simulink model "PuzzleMark5"  (R2022b)
settings: Solver=FixedStepAuto  StartTime=0.0  StopTime=160  FixedStep=0.001  RelTol=1e-3
libraries: slpidlib x2
settings Model: Creator=betel  LastModifiedBy=ivan
settings OptimizationCC: ReuseModelBlockBuffer=on

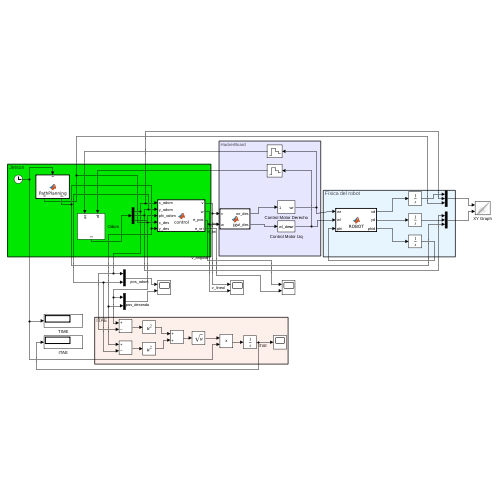
[thumbnail: Simulink's stored preview of the top-level diagram]
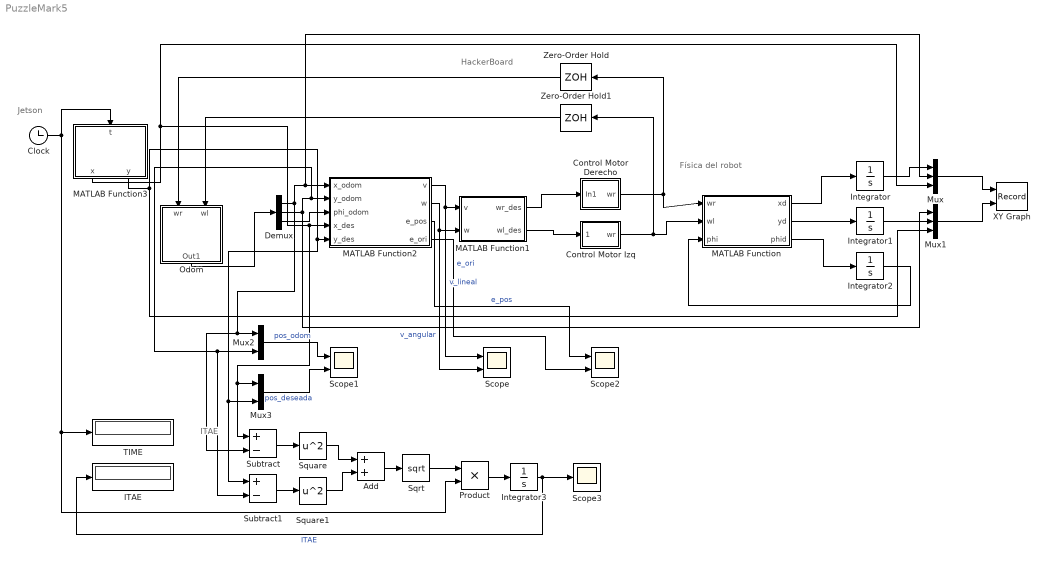
== system PuzzleMark5 ==
  note: ITAE
  note: Jetson
  note: Física del robot
  note: HackerBoard
  Add : Sum
  Clock : Clock
  Control Motor Derecho : Subsystem
  Control Motor Izq : Subsystem
  Demux : Demux  Outputs=3
  ITAE : Display
  Integrator : Integrator  ContinuousStateAttributes='x'
  Integrator1 : Integrator  ContinuousStateAttributes='y'
  Integrator2 : Integrator  ContinuousStateAttributes='orientation'
  Integrator3 : Integrator
  MATLAB Function : MATLAB Function  TreatAsAtomicUnit=on
  MATLAB Function1 : MATLAB Function  TreatAsAtomicUnit=on
  MATLAB Function2 : MATLAB Function  TreatAsAtomicUnit=on
  MATLAB Function3 : MATLAB Function  TreatAsAtomicUnit=on
  Mux : Mux  Inputs=3
  Mux1 : Mux  Inputs=3
  Mux2 : Mux  Inputs=2
  Mux3 : Mux  Inputs=2
  Odom : Subsystem
  Product : Product
  Scope : Scope  NumInputPorts=2
  Scope1 : Scope  NumInputPorts=2
  Scope2 : Scope  NumInputPorts=2
  Scope3 : Scope
  Sqrt : Sqrt
  Square : Math  Operator=square
  Square1 : Math  Operator=square
  Subtract : Sum  Inputs=+-
  Subtract1 : Sum  Inputs=+-
  TIME : Display
  XY Graph : Record  FileSettingsInternal="{\"entries\":[{\"content\":{\"excelSettings\":{\"content\":{},\"type\":\"Streamout.ExcelSettings\"}},\"type\":\"Streamout.FileSettingStorage\",\"uuid\":\"\"}],\"packageUris\":[\"http:\\/\\/schema.mathworks.com\\/mf0\\/streamout_blocks\\/R2020a\"],\"version\":\"1.0\"}"  Layout=[1 1]  SignalsInternal="{\"entries\":[{\"content\":{\"signals\":[{\"content\":{\"blockPath\":[],\"dimensions\":[3],\"domain\":\"\",\"hasChildren\":true,\"lineColor\":\"#77ac30\",\"lineWidth\":2,\"port\":1,\"signalID\":1,\"signalName\":\"Mux\"},\"type\":\"RecordBlkView.Signal\",\"uuid\":\"\"},{\"content\":{\"blockPath\":[],\"channel\":[1],\"dimensions\":[3],\"domain\":\"\",\"lineColor\":\"#139fff\",\"parentID\":1,\"plots\":[ 1 ],\"port\":1,\"signalID\":2,\"signalName\":\"Mux\"},\"type\":\"RecordBlkView.Signal\",\"uuid\":\"\"},{\"content\":{\"blockPath\":[],\"channel\":[2],\"dimensions\":[3],\"domain\":\"\",\"lineColor\":\"#64d413\",\"parentID\":1,\"plots\":[ 1 ],\"port\":1,\"signalID\":3,\"signalName\":\"Mux\"},\"type\":\"RecordBlkView.Signal\",\"uuid\":\"\"},{\"content\":{\"blockPath\":[],\"channel\":[3],\"dimensions\":[3],\"domain\":\"\",\"lineColor\":\"#4dbeee\",\"parentID\":1,\"plots\":[ 1 ],\"port\":1,\"signalID\":4,\"signalName\":\"Mux\"},\"type\":\"RecordBlkView.Signal\",\"uuid\":\"\"},{\"content\":{\"blockPath\":[],\"dimensions\":[3],\"domain\":\"\",\"hasChildren\":true,\"lineColor\":\"#a2142f\",\"lineWidth\":2,\"port\":2,\"signalID\":5,\"signalName\":\"Mux1\"},\"type\":\"RecordBlkView.Signal\",\"uuid\":\"\"},{\"content\":{\"blockPath\":[],\"channel\":[1],\"dimensions\":[3],\"domain\":\"\",\"lineColor\":\"#b746ff\",\"parentID\":5,\"plots\":[ 1 ],\"port\":2,\"signalID\":6,\"signalName\":\"Mux1\"},\"type\":\"RecordBlkView.Signal\",\"uuid\":\"\"},{\"content\":{\"blockPath\":[],\"channel\":[2],\"dimensions\":[3],\"domain\":\"\",\"lineColor\":\"#ff13a6\",\"parentID\":5,\"plots\":[ 1 ],\"port\":2,\"signalID\":7,\"signalName\":\"Mux1\"},\"type\":\"RecordBlkView.Signal\",\"uuid\":\"\"},{\"content\":{\"blockPath\":[],\"channel\":[3],\"dimensions\":[3],\"domain\":\"\",\"lineColor\":\"#fe330a\",\"parentID\":5,\"plots\":[ 1 ],\"port\":2,\"signalID\":8,\"signalName\":\"Mux1\"},\"type\":\"RecordBlkView.Signal\",\"uuid\":\"\"}]},\"type\":\"RecordBlkView.InputSignals\",\"uuid\":\"\"}],\"packageUris\":[\"http:\\/\\/schema.mathworks.com\\/mf0\\/streamout_blocks\\/R2020a\"],\"version\":\"1.0\"}"  VisualizationBindings="{\"xyplotplugin\":{\"info\":[{\"series\":[{\"bindingParametersList\":[{\"parameter\":\"X-Axis\",\"signalID\":2,\"signalName\":\"Mux(1)\"},{\"parameter\":\"Y-Axis\",\"signalID\":6,\"signalName\":\"Mux1(1)\"}],\"seriesID\":0},{\"bindingParametersList\":[{\"parameter\":\"X-Axis\",\"signalID\":3,\"signalName\":\"Mux(2)\"},{\"parameter\":\"Y-Axis\",\"signalID\":7,\"signalName\":\"Mux1(2)\"}],\"seriesID\":1},{\"bindingParametersList\":[{\"parameter\":\"X-Axis\",\"signalID\":4,\"signalName\":\"Mux(3)\"},{\"parameter\":\"Y-Axis\",\"signalID\":8,\"signalName\":\"Mux1(3)\"}],\"seriesID\":2}],\"subplotID\":1}]}}"  CompatibilityTag=XY
  Zero-Order Hold : ZeroOrderHold  SampleTime=0.01
  Zero-Order Hold1 : ZeroOrderHold  SampleTime=0.01
  wires:
  Integrator2/1 -> MATLAB Function/3(phi)
  MATLAB Function1/1(wr_des) -> Control Motor Derecho/1(In1)
  MATLAB Function2/1(v) -> Scope/1, MATLAB Function1/1(v)  "v_lineal"
  MATLAB Function2/2(w) -> Scope/2, MATLAB Function1/2(w)  "v_angular"
  MATLAB Function/1(xd) -> Integrator/1
  MATLAB Function/2(yd) -> Integrator1/1
  MATLAB Function/3(phid) -> Integrator2/1
  Odom/1(Out1) -> Demux/1
  Demux/3 -> MATLAB Function2/3(phi_odom)
  MATLAB Function1/2(wl_des) -> Control Motor Izq/1(wl_des)
  Zero-Order Hold/1 -> Odom/1(wr)
  Zero-Order Hold1/1 -> Odom/2(wl)
  Control Motor Derecho/1(wr) -> Zero-Order Hold/1, MATLAB Function/1(wr)
  Control Motor Izq/1(wr) -> Zero-Order Hold1/1, MATLAB Function/2(wl)
  Clock/1 -> Product/2, TIME/1, MATLAB Function3/1(t)
  Integrator/1 -> Mux/1
  Demux/1 -> Mux/2, MATLAB Function2/1(x_odom), Subtract/2, Mux2/1
  MATLAB Function3/1(x) -> Mux/3, Subtract/1, Mux3/1, MATLAB Function2/4(x_des)
  Mux/1 -> XY Graph/1
  Mux1/1 -> XY Graph/2
  Integrator1/1 -> Mux1/1
  Demux/2 -> Subtract1/2, Mux2/2, MATLAB Function2/2(y_odom), Mux1/2
  MATLAB Function3/2(y) -> Subtract1/1, Mux3/2, MATLAB Function2/5(y_des), Mux1/3
  Mux2/1 -> Scope1/1  "pos_odom"
  Mux3/1 -> Scope1/2  "pos_deseada"
  Subtract/1 -> Square/1
  Subtract1/1 -> Square1/1
  Square/1 -> Add/1
  Square1/1 -> Add/2
  Add/1 -> Sqrt/1
  Sqrt/1 -> Product/1
  Product/1 -> Integrator3/1
  Integrator3/1 -> ITAE/1, Scope3/1  "ITAE"
  MATLAB Function2/4(e_ori) -> Scope2/2  "e_ori"
  MATLAB Function2/3(e_pos) -> Scope2/1  "e_pos"

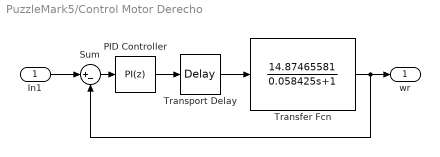
== system PuzzleMark5/Control Motor Derecho ==
  In1 : Inport
  PID Controller : slpidlib/PID Controller  Controller=PI  Form=Parallel  TimeDomain=Discrete-time  UseExternalTs=off  SampleTime=0.01  IntegratorMethod=Forward Euler  FilterMethod=Forward Euler  ControllerParametersSource=internal  P=0.03143  I=0.22281  UseKiTs=off  D=0  N=100  UseFilter=on  TunerSelectOption=Transfer Function Based (PID Tuner App)  InitialConditionSource=internal  InitialConditionForIntegrator=0  InitialConditionForFilter=0  DifferentiatorICPrevScaledInput=0  ExternalReset=none  TrackingMode=off  Kt=1  LimitOutput=on  SatLimitsSource=internal  UpperSaturationLimit=1  LowerSaturationLimit=-1  LinearizeAsGain=on  AntiWindupMode=none  Kb=1  LimitIntegrator=off  UpperIntegratorSaturationLimit=inf  LowerIntegratorSaturationLimit=-inf  POutMin=[]  POutMax=[]  IOutMin=[]  IOutMax=[]  DOutMin=[]  DOutMax=[]  NOutMin=[]  NOutMax=[]  SumOutMin=[]  SumOutMax=[]  SaturationOutMin=[]  SaturationOutMax=[]  PParamMin=[]  PParamMax=[]  IParamMin=[]  IParamMax=[]  DParamMin=[]  DParamMax=[]  NParamMin=[]  NParamMax=[]  KbParamMin=[]  KbParamMax=[]  KtParamMin=[]  KtParamMax=[]  KbOutMin=[]  KbOutMax=[]  KtOutMin=[]  KtOutMax=[]  IntegratorOutMin=[]  IntegratorOutMax=[]  FilterOutMin=[]  FilterOutMax=[]  SumI1OutMin=[]  SumI1OutMax=[]  SumI2OutMin=[]  SumI2OutMax=[]  SumI3OutMin=[]  SumI3OutMax=[]  SumI4OutMin=[]  SumI4OutMax=[]  SumDOutMin=[]  SumDOutMax=[]  DifferentiatorOutMin=[]  DifferentiatorOutMax=[]  FilterDiffOutCoefMin=[]  FilterDiffOutCoefMax=[]  ReciprocalOutMin=[]  ReciprocalOutMax=[]  SumDenOutMin=[]  SumDenOutMax=[]  SumNumOutMin=[]  SumNumOutMax=[]  DivideOutMin=[]  DivideOutMax=[]  UdiffTsProdOutMin=[]  UdiffTsProdOutMax=[]  NTsProdOutMin=[]  NTsProdOutMax=[]  UintegralTsProdOutMin=[]  UintegralTsProdOutMax=[]  UngainTsProdOutMin=[]  UngainTsProdOutMax=[]  IntegratorContinuousStateAttributes=''  IntegratorStateMustResolveToSignalObject=off  IntegratorRTWStateStorageClass=Auto  FilterContinuousStateAttributes=''  FilterStateMustResolveToSignalObject=off  FilterRTWStateStorageClass=Auto  ParallelPVariant=InternalParameters  IdealPVariant=Disabled  IVariant=InternalParameters  DVariant=Disabled  IntegratorVariant=Discrete  SatVariant=Enabled  AWVariant=Passthrough  PCopyVariant=Disabled  TRVariant=Disabled  FdbkBlocksVariant=Forward  IdealPFdbkVariant=Disabled  SatFdbkVariant=Disabled  DerivativeFilterVariant=Disabled  NVariant=Disabled  NCopyVariant=Disabled_SignalSpec  FilterICVariant=Disabled  IntegratorICVariant=InternalICs  ExternalResetVariant=Disabled  TRSumVariant=Passthrough  SumFdbkVariant=Disabled  SumVariant=Sum_PI  TsampFilterVariant=InternalTs  TsampNgainVariant=Passthrough  TsampIntegralVariant=Disabled_SignalSpec  ExternalSaturationOutDataTypeStr=Inherit: Same as second input
  Sum : Sum  Inputs=|+-
  Transfer Fcn : TransferFcn  Numerator=[14.87465581]  Denominator=[0.058425 1]
  Transport Delay : TransportDelay  DelayTime=0.043735
  wr : Outport
  wires:
  In1/1 -> Sum/1
  Sum/1 -> PID Controller/1
  Transfer Fcn/1 -> Sum/2, wr/1
  PID Controller/1 -> Transport Delay/1
  Transport Delay/1 -> Transfer Fcn/1

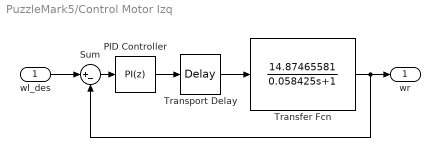
== system PuzzleMark5/Control Motor Izq ==
  wl_des : Inport
  PID Controller : slpidlib/PID Controller  Controller=PI  Form=Parallel  TimeDomain=Discrete-time  UseExternalTs=off  SampleTime=0.01  IntegratorMethod=Forward Euler  FilterMethod=Forward Euler  ControllerParametersSource=internal  P=0.03143  I=0.22281  UseKiTs=off  D=0  N=100  UseFilter=on  TunerSelectOption=Transfer Function Based (PID Tuner App)  InitialConditionSource=internal  InitialConditionForIntegrator=0  InitialConditionForFilter=0  DifferentiatorICPrevScaledInput=0  ExternalReset=none  TrackingMode=off  Kt=1  LimitOutput=on  SatLimitsSource=internal  UpperSaturationLimit=1  LowerSaturationLimit=-1  LinearizeAsGain=on  AntiWindupMode=none  Kb=1  LimitIntegrator=off  UpperIntegratorSaturationLimit=inf  LowerIntegratorSaturationLimit=-inf  POutMin=[]  POutMax=[]  IOutMin=[]  IOutMax=[]  DOutMin=[]  DOutMax=[]  NOutMin=[]  NOutMax=[]  SumOutMin=[]  SumOutMax=[]  SaturationOutMin=[]  SaturationOutMax=[]  PParamMin=[]  PParamMax=[]  IParamMin=[]  IParamMax=[]  DParamMin=[]  DParamMax=[]  NParamMin=[]  NParamMax=[]  KbParamMin=[]  KbParamMax=[]  KtParamMin=[]  KtParamMax=[]  KbOutMin=[]  KbOutMax=[]  KtOutMin=[]  KtOutMax=[]  IntegratorOutMin=[]  IntegratorOutMax=[]  FilterOutMin=[]  FilterOutMax=[]  SumI1OutMin=[]  SumI1OutMax=[]  SumI2OutMin=[]  SumI2OutMax=[]  SumI3OutMin=[]  SumI3OutMax=[]  SumI4OutMin=[]  SumI4OutMax=[]  SumDOutMin=[]  SumDOutMax=[]  DifferentiatorOutMin=[]  DifferentiatorOutMax=[]  FilterDiffOutCoefMin=[]  FilterDiffOutCoefMax=[]  ReciprocalOutMin=[]  ReciprocalOutMax=[]  SumDenOutMin=[]  SumDenOutMax=[]  SumNumOutMin=[]  SumNumOutMax=[]  DivideOutMin=[]  DivideOutMax=[]  UdiffTsProdOutMin=[]  UdiffTsProdOutMax=[]  NTsProdOutMin=[]  NTsProdOutMax=[]  UintegralTsProdOutMin=[]  UintegralTsProdOutMax=[]  UngainTsProdOutMin=[]  UngainTsProdOutMax=[]  IntegratorContinuousStateAttributes=''  IntegratorStateMustResolveToSignalObject=off  IntegratorRTWStateStorageClass=Auto  FilterContinuousStateAttributes=''  FilterStateMustResolveToSignalObject=off  FilterRTWStateStorageClass=Auto  ParallelPVariant=InternalParameters  IdealPVariant=Disabled  IVariant=InternalParameters  DVariant=Disabled  IntegratorVariant=Discrete  SatVariant=Enabled  AWVariant=Passthrough  PCopyVariant=Disabled  TRVariant=Disabled  FdbkBlocksVariant=Forward  IdealPFdbkVariant=Disabled  SatFdbkVariant=Disabled  DerivativeFilterVariant=Disabled  NVariant=Disabled  NCopyVariant=Disabled_SignalSpec  FilterICVariant=Disabled  IntegratorICVariant=InternalICs  ExternalResetVariant=Disabled  TRSumVariant=Passthrough  SumFdbkVariant=Disabled  SumVariant=Sum_PI  TsampFilterVariant=InternalTs  TsampNgainVariant=Passthrough  TsampIntegralVariant=Disabled_SignalSpec  ExternalSaturationOutDataTypeStr=Inherit: Same as second input
  Sum : Sum  Inputs=|+-
  Transfer Fcn : TransferFcn  Numerator=[14.87465581]  Denominator=[0.058425 1]
  Transport Delay : TransportDelay  DelayTime=0.043735
  wr : Outport
  wires:
  wl_des/1 -> Sum/1
  Transfer Fcn/1 -> Sum/2, wr/1
  PID Controller/1 -> Transport Delay/1
  Transport Delay/1 -> Transfer Fcn/1
  Sum/1 -> PID Controller/1

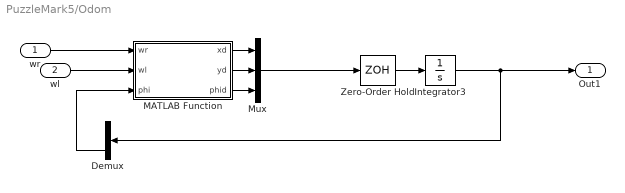
== system PuzzleMark5/Odom ==
  wr : Inport
  wl : Inport  Port=2
  Demux : Demux  Outputs=3
  Integrator3 : Integrator  InitialCondition=[0,0,0]
  MATLAB Function : MATLAB Function  TreatAsAtomicUnit=on
  Mux : Mux  Inputs=3
  Zero-Order Hold : ZeroOrderHold  SampleTime=0.1
  Out1 : Outport
  wires:
  Mux/1 -> Zero-Order Hold/1
  wl/1 -> MATLAB Function/2(wl)
  Integrator3/1 -> Demux/1, Out1/1
  Zero-Order Hold/1 -> Integrator3/1
  wr/1 -> MATLAB Function/1(wr)
  MATLAB Function/1(xd) -> Mux/1
  MATLAB Function/2(yd) -> Mux/2
  MATLAB Function/3(phid) -> Mux/3
  Demux/3 -> MATLAB Function/3(phi)

== matlab function PuzzleMark5/MATLAB Function1 ==
  data: v input; wr_des output; w input; wl_des output
function [wr_des,wl_des] = IK(v,w) %Twist local

R=0.0505;
b=0.1712;

wr_des=(v/R)+(w*b/(2*R));
wl_des=(v/R)-(w*b/(2*R));

== matlab function PuzzleMark5/MATLAB Function ==
  data: wr input; xd output; wl input; phi input; yd output; phid output
function [xd, yd, phid] = ROBOT(wr,wl,phi) %Psi es el heading.
% El heading es la orientación (dirección del mov)
% Las letras latina son translacionales, las letras griegas son
% rotacionales)
%El sufijo d significa (derivada) (Lo transforma en velocidad)

R=0.0505;%Metros
b=0.1712; %Metros

xd= (wr+wl)*(R/2)*cos(phi); %Vxl*Cos(phi)
yd= (wr+wl)*(R/2)*sin(phi); %Vxl*Sin(phi)
phid=(wr-wl)*(R/b);

== matlab function PuzzleMark5/MATLAB Function2 ==
  data: x_odom input; v output; y_odom input; phi_odom input; w output; x_des input; y_des input; e_pos output; e_ori output
%CONTROLADOR Turn and Go
function [v, w, e_pos, e_ori] = control(x_odom, y_odom, phi_odom, x_des, y_des)
 
Kl = 1.5;         % Ganancia de velocidad lineal
Kw = 2;       % Ganancia de velocidad angular

e_pos = sqrt((x_des - x_odom)^2 + (y_des - y_odom)^2);    % Error de posición
phi_des = atan2(y_des - y_odom, x_des - x_odom);          % Orientación deseada
e_ori = phi_des - phi_odom;
e_ori_norm = atan2(sin(e_ori), cos(e_ori));               % Error de orientación normalizado

% Tolerancia al error de orientación
if abs(e_ori_norm) > deg2rad(6) || e_pos < 0.05
    e_pos = 0;  % Se detiene hasta alinear o si está muy cerca
end

if abs(e_ori_norm) < 1*pi/180
    e_ori_norm = 0;
end

% Ajuste de saturaciones
v = min(e_pos * Kl, 0.1);                        % velocidad lineal
w = max(min(e_ori_norm * Kw, 0.3), -0.3);        % velocidad angular

end

%Controlador Turn while Go
% 
% function [v, w, e_pos, e_ori] = control(x_odom, y_odom, phi_odom, x_des, y_des)
% 
% Kl = 1;         % Ganancia para velocidad lineal
% Kw = 1.5;       % Ganancia para velocidad angular
% 
% % Calculo de errores
% e_pos = sqrt((x_des - x_odom)^2 + (y_des - y_odom)^2);    % Distancia al objetivo
% phi_des = atan2(y_des - y_odom, x_des - x_odom);          % Ángulo hacia el objetivo
% e_ori = phi_des - phi_odom;                               % Error angular
% e_ori_norm = atan2(sin(e_ori), cos(e_ori));               % Normalizacion
% 
% % Calculo de velocidades
% v = min(Kl * e_pos * cos(e_ori_norm), 0.1);     % Avanza más si está bien alineado
% v = max(v, 0);                                  % No retrocede
% 
% w = max(min(Kw * e_ori_norm, 0.6), -0.6);       % Corrección angular saturada
% 
% % Detenerse al estar cerca
% if e_pos < 0.05
%     v = 0;
%     w = 0;
% end
% 
% end


% % Controlador Pure-pursuit
% function [v, w] = control(x_odom, y_odom, phi_odom, x_des, y_des)
%     % Parámetros del controlador
%     L = 0.1;            % Distancia de look-ahead
%     v_max = 0.3;        % Saturación de velocidad lineal
%     w_max = 1.0;        % Saturación de velocidad angular
%     tol = 0.1;          % Tolerancia mínima de distancia al objetivo
% 
%     % Vector hacia el objetivo
%     dx = x_des - x_odom;
%     dy = y_des - y_odom;
%     distance = sqrt(dx^2 + dy^2);
% 
%     if distance > tol
%         % Ángulo hacia el objetivo
%         theta_target = atan2(dy, dx);
%         % Error angular entre orientación actual y rumbo hacia el objetivo
%         alpha = atan2(sin(theta_target - phi_odom), cos(theta_target - phi_odom));
% 
%         % Velocidad lineal: se avanza en línea recta hacia el objetivo
%         v = v_max;
% 
%         % Velocidad angular: proporcional al ángulo de giro necesario
%         w = (2 * v * sin(alpha)) / L;
%     else
%         v = 0;
%         w = 0;
%     end
% 
%     % Saturación
%     v = max(min(v, v_max), -v_max);
%     w = max(min(w, w_max), -w_max);
% end

== matlab function PuzzleMark5/Odom/MATLAB Function ==
  data: wr input; xd output; wl input; phi input; yd output; phid output
function [xd, yd, phid] = cinematica(wr,wl,phi) %Psi es el heading.
% El heading es la orientación (dirección del mov)
% Las letras latina son translacionales, las letras griegas son
% rotacionales)
%El sufijo d significa (derivada) (Lo transforma en velocidad)

R=0.0505;%Metros
b=0.1712; %Metros

xd= (wr+wl)*(R/2)*cos(phi); %Vxl*Cos(phi)
yd= (wr+wl)*(R/2)*sin(phi); %Vxl*Sin(phi)
phid=(wr-wl)*(R/b);

== matlab function PuzzleMark5/MATLAB Function3 ==
  data: x output; t input; y output
function [x, y] = PathPlanning(t)
%TRAYECTORIA DE CURVAS AMPLIAS

r = 2;             % Curvas amplias
w = 0.1 / r * 0.8;
x = r * cos(w * t) - r;
y = r * sin(w * t);


% % % %TRAYECTORIA DE CURVAS CERRADAS
% r = 0.5;             % Curvas cerradas
% w = 0.1 / r * 0.8;
% x = r * cos(w * t) - r;
% y = r * sin(w * t);


% % %TRAYECTORIA DE CUADRANTES
%     % Definir puntos objetivo (Trayectoria triangular):
%     points = [2, 3; 4, 0; 0, 0];  %Cuadrante 1
% 
%     %points = [2, -3; 4, 0; 0, 0];  %Cuadrante 2
%     %points = [-2, -3; -4, 0; 0, 0];  %Cuadrante 3
%     %points = [-2, 3; -4, 0; 0, 0];  %Cuadrante 4
% 
%     % Tiempo para permanecer en cada punto antes de cambiar (segundos)
%     hold_time = 45;
% 
%     % Determinar en qué etapa va t (cada hold_time segundos cambia de punto)
%     idx = floor(t / hold_time) + 1;
% 
%     % Asegurar que no se salga del índice
%     if idx > size(points, 1)
%         idx = size(points, 1);
%     end
% 
%     % Objetivo actual
%     x = points(idx, 1);
%     y = points(idx, 2);
% end



% % TRAYECTORIA DE ESQUINAS PRONUNCIADAS
% 
% % Parámetros del pentágono
% n_sides = 5;
% r = 2; % Radio circunscrito
% segment_duration = 20; % Tiempo por lado
% total_cycle_time = n_sides * segment_duration;
% 
% % Ángulos de los vértices (iniciando desde el vértice inferior)
% theta = linspace(-pi/2, 3*pi/2, n_sides + 1);  % -pi/2 para que el vértice inferior esté en 0,0
% x_points = r *cos(theta);
% y_points = r * sin(theta);
% 
% % Trasladar todo el pentágono para que el punto más bajo (vértice inferior) esté en (0, 0)
% x_shift = -x_points(1);
% y_shift = -y_points(1);
% x_points = x_points + x_shift;
% y_points = y_points + y_shift;
% 
% % Normalizar el tiempo para repetir la trayectoria
% t_normalized = mod(t, total_cycle_time);
% 
% % Determinar segmento actual
% segment_idx = floor(t_normalized / segment_duration) + 1;
% t_rel = t_normalized - (segment_idx - 1) * segment_duration;
% 
% % Asegurar índice dentro de rango
% if segment_idx >= length(x_points)
%     segment_idx = length(x_points) - 1;
% end
% 
% % Interpolación lineal entre puntos
% x = x_points(segment_idx) + (x_points(segment_idx+1) - x_points(segment_idx)) * (t_rel / segment_duration);
% y = y_points(segment_idx) + (y_points(segment_idx+1) - y_points(segment_idx)) * (t_rel / segment_duration);
% 
% end
